simulink model "AN_Simulink_Model_v1"  (R2019b)
settings: Solver=VariableStepAuto  StartTime=0.0  StopTime=testtime  RelTol=1e-3
InitFcn:
  | AN_InitFcn_Callback
StopFcn:
  | AN_StopFcn_Callback
values from neighbouring files (symbols this model uses):
  C1initphase = C1initphase + atan(CF/(-rzero))-atan((CF-pimag(2*i-1))/(-preal(2*i-1)))-atan((CF+pimag(2*i-1))/(-preal(2*i-1)))    [AN_Get_Model_Parameters.m]
  C1slope = 0.1    [AN_Get_Model_Parameters.m]
  C2slope = 0.2    [AN_Get_Model_Parameters.m]
  CF = 2*pi*cf    [AN_Get_Model_Parameters.m]
  cf = 1000    [AN_Set_Model_Parameters.m]
  cihc = 1    [AN_Set_Model_Parameters.m]
  fs_bilinear = 2*pi*cf/tan(2*pi*cf*tdres/2)    [AN_Get_Model_Parameters.m]
  ihcasym = 3.0    (= 3)    [AN_Get_Model_Parameters.m]
  IHCLPcoeffs = [  gainihc*c2LPihc gainihc*c2LPihc 0 1 -c1LPihc 0 ... (first row only)    [AN_Get_Model_Parameters.m]
  MEcoeffs = [m14*m11 m15*m11 m16*m11 1 m12*m11 m13*m11; m24*m21 m25*m21 m26*m21 1 m22*m21 m23*m21; m34*m31 m35*m31 m36*m31 1 m32*m31 m33*m31]    [AN_Get_Model_Parameters.m]
  MEscale = 1/megainmax    (= 0.5)    [AN_Get_Model_Parameters.m]
  norm_gainc1 = single(norm_gainc1)    [AN_Get_Model_Parameters.m]
  order_of_zero = half_order_pole    (= 5)    [AN_Get_Model_Parameters.m]
  pimag = zeros(11,1)    [AN_Get_Model_Parameters.m]
  preal = zeros(11,1)    [AN_Get_Model_Parameters.m]
  strength = (20.0e6)/(10^(corner/20))    (= 2000)    [AN_Get_Model_Parameters.m]
  tauc1 = 0.003    [AN_Get_Model_Parameters.m]
  tdres = 1/Fs    (= 2.08333333333e-05)    [AN_Set_Model_Parameters.m]
undefined symbols (not defined in the file or in its folder): bmTaumax, C2coeffs, norm_gainc2
libraries: simulink x5, dspsrcs4 x1
settings Model: NumberOfSteps=50  Creator=mblun  LastModifiedBy=t96f346
settings OptimizationCC: BlockReduction=off  ConditionallyExecuteInputs=off  DefaultParameterBehavior=Inlined
settings DebuggingCC: AlgebraicLoopMsg=error  UnderSpecifiedDimensionMsg=warning
settings HardwareCC: ProdBitPerPointer=32  ProdBitPerSizeT=32  ProdBitPerPtrDiffT=32  ProdLargestAtomicFloat=None  ProdIntDivRoundTo=Undefined  ProdEndianess=Unspecified  ProdWordSize=32  ProdHWDeviceType=ASIC/FPGA->ASIC/FPGA  TargetBitPerPointer=64  TargetBitPerSizeT=64  TargetBitPerPtrDiffT=64  TargetLongLongMode=on  TargetIntDivRoundTo=Zero  TargetEndianess=LittleEndian  TargetWordSize=64  TargetHWDeviceType=Custom Processor->MATLAB Host Computer  ProdEqTarget=off
settings SFSimCC: CustomCodeUndefinedFunction=UseInterfaceOnly

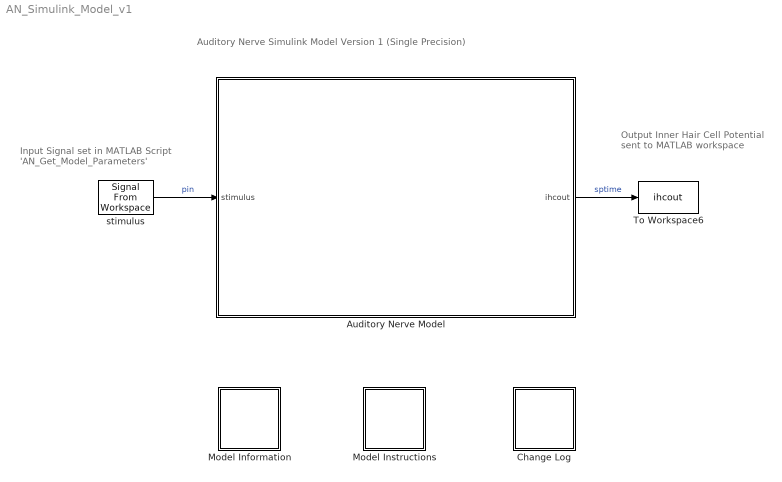
== system AN_Simulink_Model_v1 ==
  note: Input Signal set in MATLAB Script 'AN_Get_Model_Parameters'
  note: Auditory Nerve Simulink Model Version 1 (Single Precision)
  note: Output Inner Hair Cell Potential sent to MATLAB workspace
  Auditory Nerve Model : Subsystem
  Change Log : Subsystem
  Model Information : Subsystem
  Model Instructions : Subsystem
  To Workspace6 : ToWorkspace  VariableName=ihcout  SampleTime=-1
      settings: Save2DSignal=2-D array (concatenate along first dimension)
  "stimulus " : dspsrcs4/Signal From Workspace  X=RxSignal  Ts=tdres  nsamps=1  OutputAfterFinalValue=Setting to zero  ignoreOrWarnInputAndFrameLengths=off  OutputFrames=off
  wires:
  Auditory Nerve Model/1(ihcout) -> To Workspace6/1  "sptime"
  "stimulus "/1 -> Auditory Nerve Model/1(stimulus)  "pin"

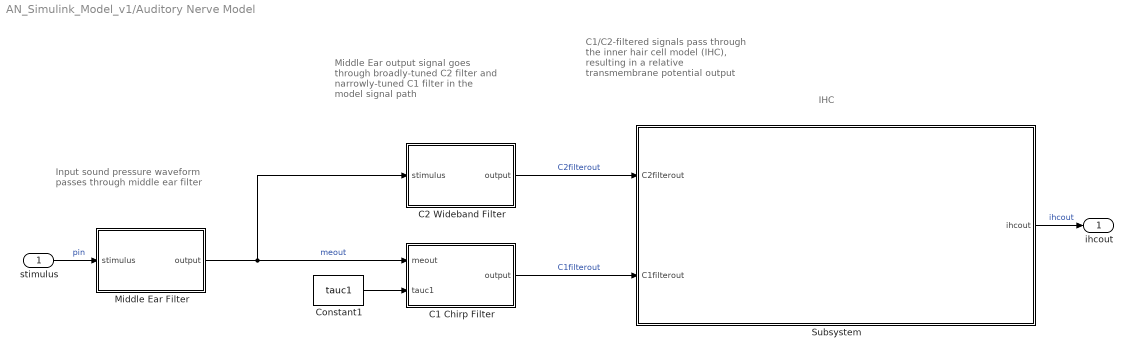
== system AN_Simulink_Model_v1/Auditory Nerve Model ==
  note: IHC
  note: Input sound pressure waveform passes through middle ear filter
  note: Middle Ear output signal goes through broadly-tuned C2 filter and narrowly-tuned C1 filter in the model signal path
  note: C1/C2-filtered signals pass through the inner hair cell model (IHC), resulting in a relative transmembrane potential output
  stimulus : Inport
  C1 Chirp Filter : Subsystem
  C2 Wideband Filter : Subsystem
  Constant1 : Constant  Value=tauc1  OutDataTypeStr=single  SampleTime=-1
  Middle Ear Filter : Subsystem
  Subsystem : Subsystem
  ihcout : Outport  VectorParamsAs1DForOutWhenUnconnected=off
  wires:
  Middle Ear Filter/1(output) -> C1 Chirp Filter/1(meout), C2 Wideband Filter/1(stimulus)  "meout"
  stimulus/1 -> Middle Ear Filter/1(stimulus)  "pin"
  C1 Chirp Filter/1(output) -> Subsystem/2(C1filterout)  "C1filterout"
  Subsystem/1(ihcout) -> ihcout/1  "ihcout"
  C2 Wideband Filter/1(output) -> Subsystem/1(C2filterout)  "C2filterout"
  Constant1/1 -> C1 Chirp Filter/2(tauc1)

== system AN_Simulink_Model_v1/Change Log ==
  Change Log : simulink/Model-Wide Utilities/Model Info  Frame=on  DisplayStringWithTags=|  HorizontalTextAlignment=Left  LeftAlignmentValue=0.02
      | The following is the change log for the AN Simulink Model. Any major version changes should be 
      | documented and summarized below.
      | 
      | ------------------------------------------------------------------------------------------------------------------------------------
      | 
      | Version 1:
      | 	
      | 	- First Draft Version of Simulink Model by Matthew Blunt --- 08/07/2019
      | 
      | ------------------------------------------------------------------------------------------------------------------------------------
      | 
      | (Next Version Here)
      | 
      | 	- (Details and Changes Here)

== system AN_Simulink_Model_v1/Model Information ==
  "Model Information " : simulink/Model-Wide Utilities/Model Info  Frame=on  DisplayStringWithTags=|  HorizontalTextAlignment=Left  LeftAlignmentValue=0.02
      | Model Name: AN_Simulink_Model_v1
      | Created By: Matthew Blunt
      | Last Modification Date: 08/07/2019
      | Most Recently Modified By: Matthew Blunt
      | Model Version: 1
      | 
      | ------------------------------------------------------------------------------------------------------------------------------------
      | 
      | Description: This is a sample-based auditory nerve Simulink model, designed to closely replicate the 
      | auditory nerve model presented in the following publication:
      | 
      | 			Bruce, I.C., Erfani, Y., and Zilany, M.S.A. (2018). "A Phenomenological
      | 			model of the synapse between the inner hair cell and auditory nerve: 
      | 			Implications of limited neurotransmitter release sites," to appear in
      | 			Hearing Research. (Special Issue on "Computational Models in Hearing".)
      | 
      | It is important to also recognize the previous iterations of the phenomenological auditory 
      | nerve model, as they served as additional references during the design of the Simulink model.
      | 
      | ------------------------------------------------------------------------------------------------------------------------------------
      | 
      | This software was developed in conjunction with Flat Earth Inc
      | 
      | Copyright 2019 Flat Earth Inc
      | 
      | THE SOFTWARE IS PROVIDED "AS IS", WITHOUT WARRANTY OF ANY KIND, EXPRESS OR
      | IMPLIED, INCLUDING BUT NOT LIMITED TO THE WARRANTIES OF MERCHANTABILITY,
      | FITNESS FOR A PARTICULAR PURPOSE AND NONINFRINGEMENT. IN NO EVENT SHALL
      | THE AUTHORS OR COPYRIGHT HOLDERS BE LIABLE FOR ANY CLAIM, DAMAGES OR
      | OTHER LIABILITY, WHETHER IN AN ACTION OF CONTRACT, TORT OR OTHERWISE,
      | ARISING FROM, OUT OF OR IN CONNECTION WITH THE SOFTWARE OR THE USE OR
      | OTHER DEALINGS IN THE SOFTWARE.
      | 
      |    		Matthew Blunt
      |   		 Flat Earth Inc
      |    		985 Technology Blvd
      |    		Bozeman, MT 59718
      |    		support@flatearthinc.com

== system AN_Simulink_Model_v1/Model Instructions ==
  "Model Instructions " : simulink/Model-Wide Utilities/Model Info  Frame=on  DisplayStringWithTags=|  HorizontalTextAlignment=Left  LeftAlignmentValue=0.02
      | The following is a full set of instructions outlining the necessary steps to be taken in order to run the 
      | AN Simulink Model. Instructions can also be found in the readme file found in the
      | AN_Simulink_Model_v1_Doubles folder.
      | 
      | ------------------------------------------------------------------------------------------------------------------------------------
      | 
      | ** Quick Start Instructions **
      | 
      | If the user desires to simply run the model as is, refer to the Quick Start
      | Instructions pdf, which gives a quick visual tutorial on running the Auditory
      | Nerve Simulink Model.
      | 
      | ------------------------------------------------------------------------------------------------------------------------------------
      | 
      | ** Modify Model Instructions **
      | 
      | If the user desires to make modifications to the model before runtime,
      | refer to the Modify Model Instructions pdf, which gives a quick visual
      | tutorial on modifying the Auditory Nerve Simulink Model.
      | 
      | ------------------------------------------------------------------------------------------------------------------------------------
      | 
      | ** Verify Model Instructions **
      | 
      | If the user desires to verify model functionality against the original 
      | model source code, instructions are listed below, as well as in the readme.txt file
      | 
      | 1. Make sure MATLAB R2019a and a compatible C compiler are downloaded on the
      | machine the model will be running on. The C compiler is needed for C functions
      | used in the test/verification process. The compiler used for testing was the
      | MinGW-w64 C/C++ Compiler. This can be easily accessed for free in the Add-On
      | Explorer found in the MATLAB home tab.
      | 
      | 2. Open the AN_Simulink_Model_v1_Doubles folder in MATLAB. This is necessary in
      | order for the Simulink model to interact with MATLAB.
      | 
      | 3. Edit model parameters, if necessary. This can be done by adjusting the
      | overall model parameters set in the AN_Set_Model_Parameters script, or adjusting
      | other parameters in the AN_Get_Model_Parameters script. Both scripts are found
      | in the AN_Simulink_Model_v1_Doubles folder.
      | 
      | 4. Set the 'verificationflag' boolean to 'true' in the AN_Set_Model_Parameters
      | script. This enables the model to run the comparison C/MATLAB source functions
      | which are compared to the Simulink Model.
      | 
      | 5. Run the model. This is done by simply clicking the green 'Run' button
      | located at the top panel of Simulink. In addition, the model can be stepped
      | through in increments, using the 'Step Through' button to the right of the
      | 'Run' button.

== system AN_Simulink_Model_v1/Auditory Nerve Model/C1 Chirp Filter ==
  note: C1 Chirp Filter:
      |
      | Inputs : ME Filtered Signal (meout)
      | C1 Coefficients (a&b)
      | Normalizing Gain (norm_gain)
      |
      | Output : C1 Filtered Signal (c1filterout)
      |
      | - 10th Order IIR Bandpass Filter
      |
      | - Coefficients are determined in previous Get C1 Coefficients block
      |
      | - Implemented w/ Simulink biquad block
  note: Get C1 Coefficients
      |
      | Input : Pole-Shifting Feedback Parameter (rsigma)
      |
      | Outputs : C1 Coefficients (a&b)
      | Normalizing Gain (norm_gain)
      |
      | - Consists of various calculations to shift continuous-time pole locations according to rsigma feedback, then apply a bilinear transformation to bring the poles to the digital space before finding the coefficients for the C1 filter
  note: Calculate C1 Filter Output
      |
      | - Simply scale the output by cihc
  note: Calculate Pole-Shifting Parameter rsigma
      |
      | Input : C1 Feedback Time Constant (tauc1)
      |
      | Outputs : Pole-Shifting Parameter rsigma
      |
      | - Simple calculation to find rsigma from time constant feedback input
  meout : Inport
  tauc1 : Inport  Port=2
  C1 FIlter : Subsystem
  Calculate C1filterout : Subsystem
  Calculate rsigma : Subsystem
  Get C1 Coefficients : Subsystem
  output : Outport  VectorParamsAs1DForOutWhenUnconnected=off
  wires:
  meout/1 -> C1 FIlter/1(meout)
  C1 FIlter/1(Out1) -> Calculate C1filterout/1(C1filterouttmp)  "c1filterouttmp"
  Get C1 Coefficients/1(b0(5)) -> C1 FIlter/2(b0(5))
  Get C1 Coefficients/2(b0(3)) -> C1 FIlter/3(b0(3))
  Get C1 Coefficients/3(b0(1)) -> C1 FIlter/4(b0(1))
  Get C1 Coefficients/4(b1(5)) -> C1 FIlter/5(b1(5))
  Get C1 Coefficients/5(b1(3)) -> C1 FIlter/6(b1(3))
  Get C1 Coefficients/6(b1(1)) -> C1 FIlter/7(b1(1))
  Get C1 Coefficients/7(b2(5)) -> C1 FIlter/8(b2(5))
  Get C1 Coefficients/8(b2(3)) -> C1 FIlter/9(b2(3))
  Get C1 Coefficients/9(b2(1)) -> C1 FIlter/10(b2(1))
  Get C1 Coefficients/10(a2(5)) -> C1 FIlter/11(a2(5))
  Get C1 Coefficients/11(a2(3)) -> C1 FIlter/12(a2(3))
  Get C1 Coefficients/12(a2(1)) -> C1 FIlter/13(a2(1))
  Get C1 Coefficients/13(a1(1)) -> C1 FIlter/14(a1(1))
  Get C1 Coefficients/14(a1(3)) -> C1 FIlter/15(a1(3))
  Get C1 Coefficients/15(a1(5)) -> C1 FIlter/16(a1(5))
  Calculate C1filterout/1(C1filterout) -> output/1  "C1filterout"
  Calculate rsigma/1(rsigma) -> Get C1 Coefficients/1(rsigma)  "rsigma"
  tauc1/1 -> Calculate rsigma/1(tauc1)  "tauc1"

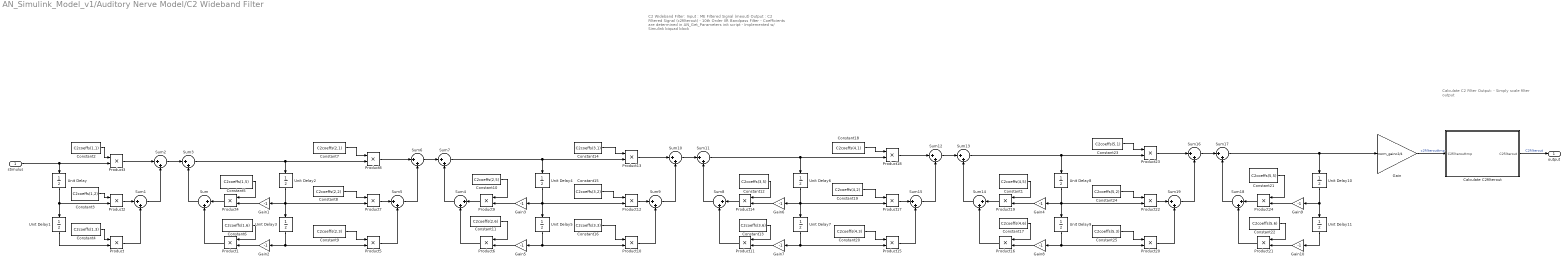
== system AN_Simulink_Model_v1/Auditory Nerve Model/C2 Wideband Filter ==
  note: C2 Wideband Filter:
      |
      | Input : ME Filtered Signal (meout)
      |
      | Output : C2 Filtered Signal (c2filterout)
      |
      | - 10th Order IIR Bandpass Filter
      |
      | - Coefficients are determined in AN_Get_Parameters init script
      |
      | - Implemented w/ Simulink biquad block
  note: Calculate C2 Filter Output:
      |
      | - Simply scale filter output
  stimulus : Inport
  Calculate C2filterout : Subsystem
  Constant1 : Constant  Value=C2coeffs(4,5)  OutDataTypeStr=single  SampleTime=-1
  Constant10 : Constant  Value=C2coeffs(2,5)  OutDataTypeStr=single  SampleTime=-1
  Constant11 : Constant  Value=C2coeffs(2,6)  OutDataTypeStr=single  SampleTime=-1
  Constant12 : Constant  Value=C2coeffs(3,5)  OutDataTypeStr=single  SampleTime=-1
  Constant13 : Constant  Value=C2coeffs(3,6)  OutDataTypeStr=single  SampleTime=-1
  Constant14 : Constant  Value=C2coeffs(3,1)  OutDataTypeStr=single  SampleTime=-1
  Constant15 : Constant  Value=C2coeffs(3,2)  OutDataTypeStr=single  SampleTime=-1
  Constant16 : Constant  Value=C2coeffs(3,3)  OutDataTypeStr=single  SampleTime=-1
  Constant17 : Constant  Value=C2coeffs(4,6)  OutDataTypeStr=single  SampleTime=-1
  Constant18 : Constant  Value=C2coeffs(4,1)  OutDataTypeStr=single  SampleTime=-1
  Constant19 : Constant  Value=C2coeffs(4,2)  OutDataTypeStr=single  SampleTime=-1
  Constant2 : Constant  Value=C2coeffs(1,1)  OutDataTypeStr=single  SampleTime=-1
  Constant20 : Constant  Value=C2coeffs(4,3)  OutDataTypeStr=single  SampleTime=-1
  Constant21 : Constant  Value=C2coeffs(5,5)  OutDataTypeStr=single  SampleTime=-1
  Constant22 : Constant  Value=C2coeffs(5,6)  OutDataTypeStr=single  SampleTime=-1
  Constant23 : Constant  Value=C2coeffs(5,1)  OutDataTypeStr=single  SampleTime=-1
  Constant24 : Constant  Value=C2coeffs(5,2)  OutDataTypeStr=single  SampleTime=-1
  Constant25 : Constant  Value=C2coeffs(5,3)  OutDataTypeStr=single  SampleTime=-1
  Constant3 : Constant  Value=C2coeffs(1,2)  OutDataTypeStr=single  SampleTime=-1
  Constant4 : Constant  Value=C2coeffs(1,3)  OutDataTypeStr=single  SampleTime=-1
  Constant5 : Constant  Value=C2coeffs(1,5)  OutDataTypeStr=single  SampleTime=-1
  Constant6 : Constant  Value=C2coeffs(1,6)  OutDataTypeStr=single  SampleTime=-1
  Constant7 : Constant  Value=C2coeffs(2,1)  OutDataTypeStr=single  SampleTime=-1
  Constant8 : Constant  Value=C2coeffs(2,2)  OutDataTypeStr=single  SampleTime=-1
  Constant9 : Constant  Value=C2coeffs(2,3)  OutDataTypeStr=single  SampleTime=-1
  Gain : Gain  Gain=norm_gainc2/4
  Gain{1..10} (10 alike) : Gain  Gain=-1
  Product{,1..24} (25 alike) : Product
  Sum{,1..19} (20 alike) : Sum  Inputs=|++
  Unit Delay{,1..11} (12 alike) : UnitDelay  SampleTime=-1  HasFrameUpgradeWarning=on
  output : Outport  VectorParamsAs1DForOutWhenUnconnected=off
  wires:
  Sum17/1 -> Gain/1, Unit Delay10/1
  Gain/1 -> Calculate C2filterout/1(C2filterouttmp)  "c2filterouttmp"
  Calculate C2filterout/1(C2filterout) -> output/1  "C2filterout"
  Sum8/1 -> Sum11/2
  Gain4/1 -> Product19/2
  Sum10/1 -> Sum11/1
  Constant15/1 -> Product12/1
  Unit Delay10/1 -> Unit Delay11/1, Gain9/1
  Product17/1 -> Sum15/1
  Constant6/1 -> Product1/1
  Constant22/1 -> Product21/1
  Unit Delay6/1 -> Product17/2, Unit Delay7/1, Gain6/1
  Sum11/1 -> Unit Delay6/1, Product18/2
  Sum6/1 -> Sum7/1
  Product18/1 -> Sum12/1
  Product23/1 -> Sum16/1
  Constant21/1 -> Product24/1
  Unit Delay8/1 -> Product22/2, Unit Delay9/1, Gain4/1
  Gain3/1 -> Product9/2
  Constant19/1 -> Product17/1
  Product/1 -> Sum1/2
  Unit Delay/1 -> Unit Delay1/1, Product2/2
  Product20/1 -> Sum19/2
  Sum3/1 -> Unit Delay2/1, Product8/2
  Gain2/1 -> Product1/2
  Constant5/1 -> Product4/1
  Constant12/1 -> Product14/1
  Sum15/1 -> Sum12/2
  Sum4/1 -> Sum7/2
  Constant14/1 -> Product13/1
  Constant10/1 -> Product9/1
  Sum14/1 -> Sum13/2
  Unit Delay11/1 -> Gain10/1
  Product13/1 -> Sum10/1
  Product4/1 -> Sum/1
  Gain10/1 -> Product21/2
  Constant8/1 -> Product7/1
  Sum2/1 -> Sum3/1
  Constant4/1 -> Product/1
  Sum7/1 -> Unit Delay4/1, Product13/2
  Unit Delay7/1 -> Product15/2, Gain7/1
  Sum12/1 -> Sum13/1
  Unit Delay9/1 -> Product20/2, Gain8/1
  Product1/1 -> Sum/2
  Sum18/1 -> Sum17/2
  Sum1/1 -> Sum2/2
  Constant23/1 -> Product23/1
  Product24/1 -> Sum18/1
  Product11/1 -> Sum8/2
  Product21/1 -> Sum18/2
  Constant3/1 -> Product2/1
  Constant2/1 -> Product3/1
  Product5/1 -> Sum5/2
  Constant7/1 -> Product8/1
  Sum/1 -> Sum3/2
  Product8/1 -> Sum6/1
  Gain5/1 -> Product6/2
  Gain9/1 -> Product24/2
  Product16/1 -> Sum14/2
  Unit Delay4/1 -> Product12/2, Unit Delay5/1, Gain3/1
  Constant16/1 -> Product10/1
  Product15/1 -> Sum15/2
  Constant20/1 -> Product15/1
  stimulus/1 -> Product3/2, Unit Delay/1
  Product3/1 -> Sum2/1
  Unit Delay1/1 -> Product/2
  Product2/1 -> Sum1/1
  Constant24/1 -> Product22/1
  Gain8/1 -> Product16/2
  Sum16/1 -> Sum17/1
  Unit Delay3/1 -> Product5/2, Gain2/1
  Constant9/1 -> Product5/1
  Product6/1 -> Sum4/2
  Sum19/1 -> Sum16/2
  Gain1/1 -> Product4/2
  Product10/1 -> Sum9/2
  Product22/1 -> Sum19/1
  Unit Delay5/1 -> Product10/2, Gain5/1
  Unit Delay2/1 -> Product7/2, Unit Delay3/1, Gain1/1
  Product9/1 -> Sum4/1
  Gain6/1 -> Product14/2
  Constant1/1 -> Product19/1
  Constant17/1 -> Product16/1
  Product14/1 -> Sum8/1
  Product19/1 -> Sum14/1
  Product7/1 -> Sum5/1
  Constant13/1 -> Product11/1
  Constant25/1 -> Product20/1
  Gain7/1 -> Product11/2
  Constant11/1 -> Product6/1
  Sum5/1 -> Sum6/2
  Constant18/1 -> Product18/1
  Sum13/1 -> Unit Delay8/1, Product23/2
  Sum9/1 -> Sum10/2
  Product12/1 -> Sum9/1

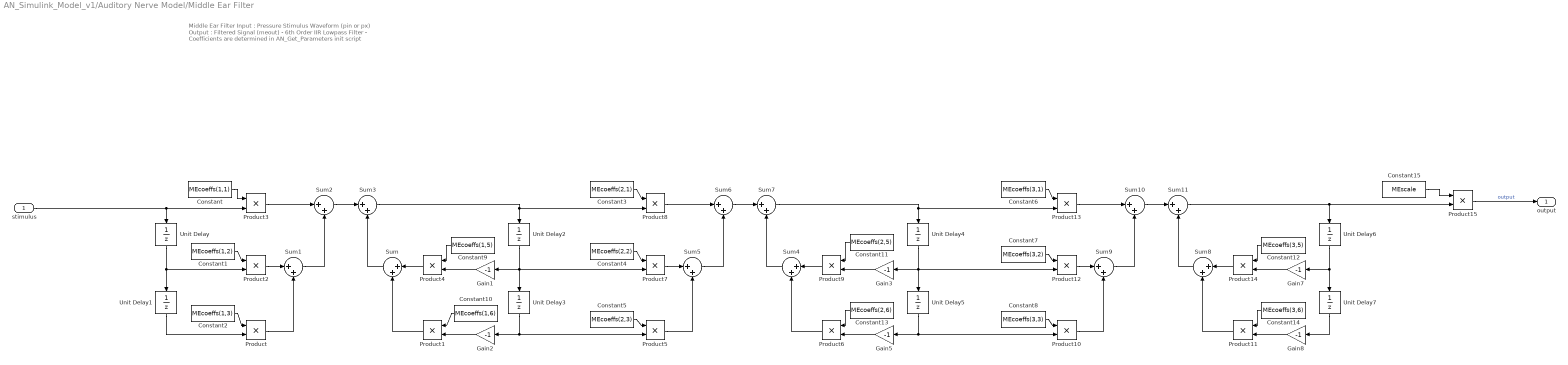
== system AN_Simulink_Model_v1/Auditory Nerve Model/Middle Ear Filter ==
  note: Middle Ear Filter
      |
      | Input : Pressure Stimulus Waveform (pin or px)
      |
      | Output : Filtered Signal (meout)
      |
      | - 6th Order IIR Lowpass Filter
      |
      | - Coefficients are determined in AN_Get_Parameters init script
  stimulus : Inport
  Constant : Constant  Value=MEcoeffs(1,1)  OutDataTypeStr=single  SampleTime=-1
  Constant1 : Constant  Value=MEcoeffs(1,2)  OutDataTypeStr=single  SampleTime=-1
  Constant10 : Constant  Value=MEcoeffs(1,6)  OutDataTypeStr=single  SampleTime=-1
  Constant11 : Constant  Value=MEcoeffs(2,5)  OutDataTypeStr=single  SampleTime=-1
  Constant12 : Constant  Value=MEcoeffs(3,5)  OutDataTypeStr=single  SampleTime=-1
  Constant13 : Constant  Value=MEcoeffs(2,6)  OutDataTypeStr=single  SampleTime=-1
  Constant14 : Constant  Value=MEcoeffs(3,6)  OutDataTypeStr=single  SampleTime=-1
  Constant15 : Constant  Value=MEscale  OutDataTypeStr=single  SampleTime=-1
  Constant2 : Constant  Value=MEcoeffs(1,3)  OutDataTypeStr=single  SampleTime=-1
  Constant3 : Constant  Value=MEcoeffs(2,1)  OutDataTypeStr=single  SampleTime=-1
  Constant4 : Constant  Value=MEcoeffs(2,2)  OutDataTypeStr=single  SampleTime=-1
  Constant5 : Constant  Value=MEcoeffs(2,3)  OutDataTypeStr=single  SampleTime=-1
  Constant6 : Constant  Value=MEcoeffs(3,1)  OutDataTypeStr=single  SampleTime=-1
  Constant7 : Constant  Value=MEcoeffs(3,2)  OutDataTypeStr=single  SampleTime=-1
  Constant8 : Constant  Value=MEcoeffs(3,3)  OutDataTypeStr=single  SampleTime=-1
  Constant9 : Constant  Value=MEcoeffs(1,5)  OutDataTypeStr=single  SampleTime=-1
  Gain{1..3,5,7..8} (6 alike) : Gain  Gain=-1
  Product{,1..15} (16 alike) : Product
  Sum{,1..11} (12 alike) : Sum  Inputs=|++
  Unit Delay{,1..7} (8 alike) : UnitDelay  SampleTime=-1  HasFrameUpgradeWarning=on
  output : Outport  VectorParamsAs1DForOutWhenUnconnected=off
  wires:
  Product15/1 -> output/1  "output"
  Constant13/1 -> Product6/1
  Constant6/1 -> Product13/1
  Gain8/1 -> Product11/2
  Sum8/1 -> Sum11/2
  Constant11/1 -> Product9/1
  Sum9/1 -> Sum10/2
  Constant12/1 -> Product14/1
  Constant15/1 -> Product15/1
  Constant14/1 -> Product11/1
  Unit Delay5/1 -> Product10/2, Gain5/1
  Sum4/1 -> Sum7/2
  Unit Delay/1 -> Unit Delay1/1, Product2/2
  Constant4/1 -> Product7/1
  Unit Delay7/1 -> Gain8/1
  Constant8/1 -> Product10/1
  Sum/1 -> Sum3/2
  Constant2/1 -> Product/1
  Constant7/1 -> Product12/1
  Product10/1 -> Sum9/2
  Constant/1 -> Product3/1
  Sum7/1 -> Product13/2, Unit Delay4/1
  Product1/1 -> Sum/2
  Product7/1 -> Sum5/1
  Constant1/1 -> Product2/1
  Unit Delay1/1 -> Product/2
  Product14/1 -> Sum8/1
  Gain7/1 -> Product14/2
  Sum3/1 -> Product8/2, Unit Delay2/1
  Product11/1 -> Sum8/2
  Sum5/1 -> Sum6/2
  stimulus/1 -> Product3/2, Unit Delay/1
  Sum1/1 -> Sum2/2
  Product6/1 -> Sum4/2
  Product12/1 -> Sum9/1
  Product5/1 -> Sum5/2
  Product3/1 -> Sum2/1
  Product2/1 -> Sum1/1
  Product9/1 -> Sum4/1
  Unit Delay6/1 -> Unit Delay7/1, Gain7/1
  Unit Delay3/1 -> Product5/2, Gain2/1
  Product13/1 -> Sum10/1
  Product4/1 -> Sum/1
  Unit Delay4/1 -> Product12/2, Unit Delay5/1, Gain3/1
  Product/1 -> Sum1/2
  Constant5/1 -> Product5/1
  Sum11/1 -> Product15/2, Unit Delay6/1
  Unit Delay2/1 -> Product7/2, Unit Delay3/1, Gain1/1
  Product8/1 -> Sum6/1
  Gain2/1 -> Product1/2
  Sum10/1 -> Sum11/1
  Sum6/1 -> Sum7/1
  Constant9/1 -> Product4/1
  Constant10/1 -> Product1/1
  Sum2/1 -> Sum3/1
  Gain1/1 -> Product4/2
  Gain3/1 -> Product9/2
  Gain5/1 -> Product6/2
  Constant3/1 -> Product8/1

== system AN_Simulink_Model_v1/Auditory Nerve Model/Subsystem ==
  note: Sum Nonlinear Function Outputs
  note: IHC C2 Nonlinear Logarithmic Transduction Function
      |
      | Input : C2 Filtered Signal (c2filterout)
      |
      | Output : C2 Transduction Function Output (c2vihctmp)
  note: IHC C1 Nonlinear Logarithmic Transduction Function
      |
      | Input : C1 Filtered Signal (c1filterout)
      |
      | Output : C1 Transduction Function Output (c1vihctmp)
  note: IHC Lowpass Filter
      |
      | Input : Sum of C1 and C2 Nonlinear Outputs (ihcnonlinout)
      |
      | Output : IHC Output (ihcout)
      |
      | - 7th Order IIR Lowpass Filter
      |
      | - Implemented using Simulink biquad
  C2filterout : Inport
  C1filterout : Inport  Port=2
  IHC C1 NL Logarithmic Function : Subsystem
  IHC C2 NL Logarithmic Function : Subsystem
  IHC LP Filter : Subsystem
  Sum1 : Sum  Inputs=|++
  ihcout : Outport  VectorParamsAs1DForOutWhenUnconnected=off
  wires:
  IHC C2 NL Logarithmic Function/1(output) -> Sum1/1  "c2vihctmp"
  IHC C1 NL Logarithmic Function/1(output) -> Sum1/2  "c1vihctmp"
  C1filterout/1 -> IHC C1 NL Logarithmic Function/1(stimulus)  "c1filterout"
  IHC LP Filter/1(output) -> ihcout/1  "ihcout"
  Sum1/1 -> IHC LP Filter/1(stimulus)  "ihcnonlinout"
  C2filterout/1 -> IHC C2 NL Logarithmic Function/1(stimulus)  "c2filterout"

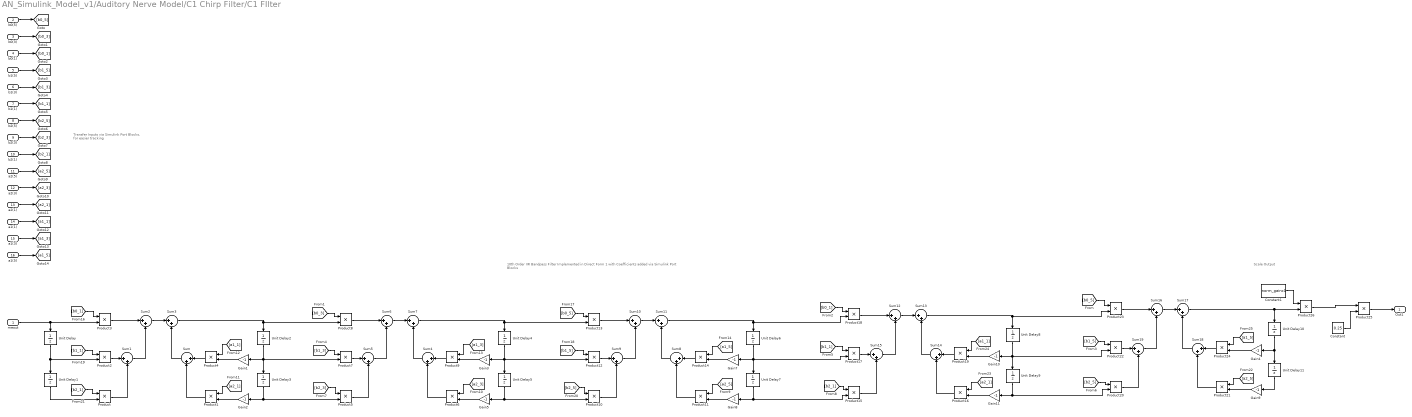
== system AN_Simulink_Model_v1/Auditory Nerve Model/C1 Chirp Filter/C1 FIlter ==
  note: Transfer Inputs via Simulink Port Blocks, for easier tracking
  note: 10th Order IIR Bandpass Filter Implemented in Direct Form 1 with Coefficients added via Simulink Port Blocks
  note: Scale Output
  meout : Inport
  b0(5) : Inport  Port=2
  b0(3) : Inport  Port=3
  b0(1) : Inport  Port=4
  b1(5) : Inport  Port=5
  b1(3) : Inport  Port=6
  b1(1) : Inport  Port=7
  b2(5) : Inport  Port=8
  b2(3) : Inport  Port=9
  b2(1) : Inport  Port=10
  a2(5) : Inport  Port=11
  a2(3) : Inport  Port=12
  a2(1) : Inport  Port=13
  a1(1) : Inport  Port=14
  a1(3) : Inport  Port=15
  a1(5) : Inport  Port=16
  Constant : Constant  Value=0.25  OutDataTypeStr=single  SampleTime=-1
  Constant1 : Constant  Value=norm_gainc1  OutDataTypeStr=single  SampleTime=-1
  Gain{1..5,7..11} (10 alike) : Gain  Gain=-1
  Product{,1..24} (25 alike) : Product
  Product25 : Product  OutDataTypeStr=single
  Product26 : Product  OutDataTypeStr=single
  Sum{,1..19} (20 alike) : Sum  Inputs=|++
  Unit Delay{,1..11} (12 alike) : UnitDelay  SampleTime=-1  HasFrameUpgradeWarning=on
  Out1 : Outport  VectorParamsAs1DForOutWhenUnconnected=off
  wires:
  [a1_5] -> Product14/1
  Product15/1 -> Sum15/2
  Product16/1 -> Sum14/2
  Sum5/1 -> Sum6/2
  Sum15/1 -> Sum12/2
  Unit Delay2/1 -> Product7/2, Unit Delay3/1, Gain1/1
  Unit Delay6/1 -> Product17/2, Unit Delay7/1, Gain7/1
  [b1_3] -> Product7/1
  Sum1/1 -> Sum2/2
  [b0_1] -> Product3/1
  Product4/1 -> Sum/1
  Unit Delay8/1 -> Product22/2, Unit Delay9/1, Gain10/1
  Product12/1 -> Sum9/1
  Sum17/1 -> Product26/2, Unit Delay10/1
  Product3/1 -> Sum2/1
  [b2_3] -> Product5/1
  Sum7/1 -> Product13/2, Unit Delay4/1
  [a2_1] -> Product1/1
  [b2_1] -> Product/1
  Product24/1 -> Sum18/1
  Unit Delay3/1 -> Product5/2, Gain2/1
  Product5/1 -> Sum5/2
  Unit Delay4/1 -> Product12/2, Unit Delay5/1, Gain3/1
  Sum13/1 -> Product23/2, Unit Delay8/1
  Sum3/1 -> Product8/2, Unit Delay2/1
  Sum4/1 -> Sum7/2
  Product19/1 -> Sum14/1
  Product7/1 -> Sum5/1
  Product10/1 -> Sum9/2
  Product20/1 -> Sum19/2
  [a1_5] -> Product24/1
  Sum6/1 -> Sum7/1
  [b0_5] -> Product13/1
  [a1_3] -> Product9/1
  Product22/1 -> Sum19/1
  Product8/1 -> Sum6/1
  meout/1 -> Product3/2, Unit Delay/1
  Product2/1 -> Sum1/1
  Sum11/1 -> Product18/2, Unit Delay6/1
  Unit Delay5/1 -> Product10/2, Gain5/1
  [b1_5] -> Product12/1
  Sum2/1 -> Sum3/1
  Product11/1 -> Sum8/2
  Sum19/1 -> Sum16/2
  [b2_5] -> Product20/1
  Product14/1 -> Sum8/1
  Product18/1 -> Sum12/1
  Sum8/1 -> Sum11/2
  [b0_3] -> Product8/1
  Sum12/1 -> Sum13/1
  [b0_5] -> Product23/1
  [b0_1] -> Product18/1
  [a1_1] -> Product19/1
  [a2_5] -> Product21/1
  Unit Delay/1 -> Unit Delay1/1, Product2/2
  Product17/1 -> Sum15/1
  Unit Delay7/1 -> Product15/2, Gain8/1
  Unit Delay10/1 -> Unit Delay11/1, Gain4/1
  [a2_5] -> Product11/1
  Unit Delay11/1 -> Gain9/1
  Product25/1 -> Out1/1
  Product23/1 -> Sum16/1
  Product9/1 -> Sum4/1
  [b1_1] -> Product17/1
  Product13/1 -> Sum10/1
  Product6/1 -> Sum4/2
  Sum9/1 -> Sum10/2
  Sum16/1 -> Sum17/1
  Product21/1 -> Sum18/2
  [b1_1] -> Product2/1
  Sum18/1 -> Sum17/2
  [b1_5] -> Product22/1
  [a2_1] -> Product16/1
  [a2_3] -> Product6/1
  Sum10/1 -> Sum11/1
  [b2_5] -> Product10/1
  [b2_1] -> Product15/1
  Product/1 -> Sum1/2
  Unit Delay9/1 -> Product20/2, Gain11/1
  Sum14/1 -> Sum13/2
  [a1_1] -> Product4/1
  Sum/1 -> Sum3/2
  Unit Delay1/1 -> Product/2
  Product1/1 -> Sum/2
  b0(5)/1 -> [b0_5]
  b0(3)/1 -> [b0_3]
  b0(1)/1 -> [b0_1]
  b1(5)/1 -> [b1_5]
  b1(3)/1 -> [b1_3]
  b1(1)/1 -> [b1_1]
  b2(5)/1 -> [b2_5]
  b2(3)/1 -> [b2_3]
  b2(1)/1 -> [b2_1]
  a2(5)/1 -> [a2_5]
  a2(3)/1 -> [a2_3]
  a2(1)/1 -> [a2_1]
  a1(1)/1 -> [a1_1]
  a1(3)/1 -> [a1_3]
  a1(5)/1 -> [a1_5]
  Gain1/1 -> Product4/2
  Gain2/1 -> Product1/2
  Gain3/1 -> Product9/2
  Gain5/1 -> Product6/2
  Gain7/1 -> Product14/2
  Gain8/1 -> Product11/2
  Gain10/1 -> Product19/2
  Gain11/1 -> Product16/2
  Gain4/1 -> Product24/2
  Gain9/1 -> Product21/2
  Constant/1 -> Product25/2
  Product26/1 -> Product25/1
  Constant1/1 -> Product26/1

== system AN_Simulink_Model_v1/Auditory Nerve Model/C1 Chirp Filter/Calculate C1filterout ==
  C1filterouttmp : Inport
  Gain1 : Gain  Gain=cihc
  C1filterout : Outport  VectorParamsAs1DForOutWhenUnconnected=off
  wires:
  C1filterouttmp/1 -> Gain1/1
  Gain1/1 -> C1filterout/1

== system AN_Simulink_Model_v1/Auditory Nerve Model/C1 Chirp Filter/Calculate rsigma ==
  note: Note: There are multiple HDL-friendly recipricol blocks. Use this block type for highest accuracy.
  note: Calculating rsigma using time constant feedback input
  tauc1 : Inport
  Constant2 : Constant  Value=bmTaumax  OutDataTypeStr=single  SampleTime=-1
  Reciprocal : Product  Inputs=/  SaturateOnIntegerOverflow=on  RndMeth=Zero
  Reciprocal1 : Product  Inputs=/  SaturateOnIntegerOverflow=on  RndMeth=Zero
  Subtract : Sum  Inputs=+-
  rsigma : Outport  VectorParamsAs1DForOutWhenUnconnected=off
  wires:
  tauc1/1 -> Reciprocal/1
  Constant2/1 -> Reciprocal1/1
  Reciprocal/1 -> Subtract/1
  Reciprocal1/1 -> Subtract/2
  Subtract/1 -> rsigma/1

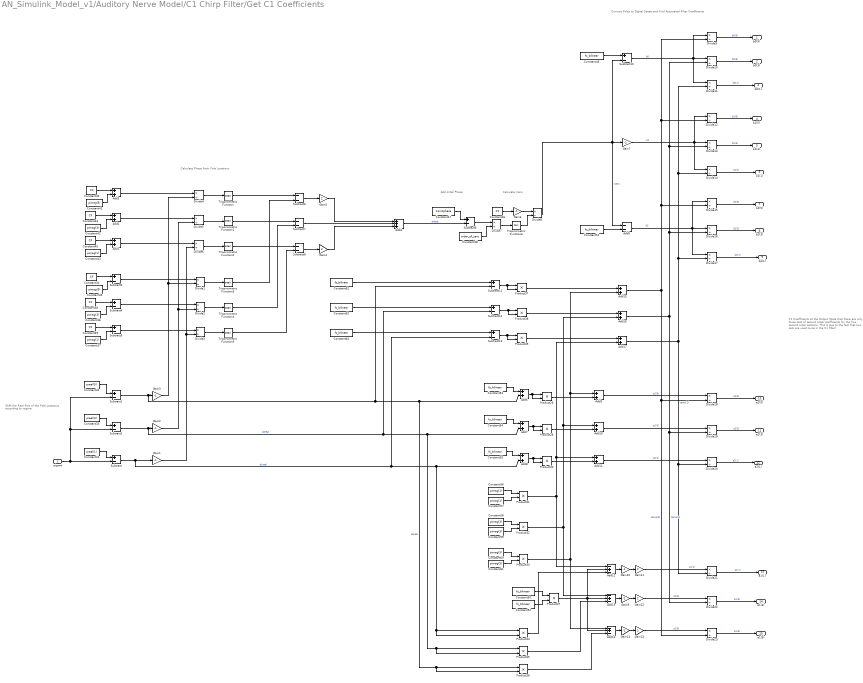
== system AN_Simulink_Model_v1/Auditory Nerve Model/C1 Chirp Filter/Get C1 Coefficients ==
  note: Calculate Phase from Pole Locations
  note: Shift the Real Part of the Pole Locations according to rsigma
  note: Add Initial Phase
  note: Calculate rzero
  note: Convert Poles to Digital Spcae and Find Associated Filter Coefficients
  note: C1 Coefficients at the Output (Note that there are only three sets of second order coefficients for the five second order sections. This is due to the fact that two sets are used twice in the C1 filter)
  rsigma : Inport
  Add{1..3,6..11,15..17} (12 alike) : Sum
  Add12 : Sum  Inputs=-+-
  Add13 : Sum  Inputs=-+-
  Add14 : Sum  Inputs=-+-
  Add4 : Sum  Inputs=+++
  Add5 : Sum  Inputs=--
  Constant31 : Constant  Value=preal(1)  OutDataTypeStr=single  SampleTime=-1
  Constant32 : Constant  Value=preal(5)  OutDataTypeStr=single  SampleTime=-1
  Constant33 : Constant  Value=preal(3)  OutDataTypeStr=single  SampleTime=-1
  Constant{34,38..40,44..46} (7 alike) : Constant  Value=CF  OutDataTypeStr=single  SampleTime=-1
  Constant{35,41,60..61} (4 alike) : Constant  Value=pimag(5)  OutDataTypeStr=single  SampleTime=-1
  Constant{36,42,58..59} (4 alike) : Constant  Value=pimag(3)  OutDataTypeStr=single  SampleTime=-1
  Constant{37,43,56..57} (4 alike) : Constant  Value=pimag(1)  OutDataTypeStr=single  SampleTime=-1
  Constant47 : Constant  Value=C1initphase  OutDataTypeStr=single  SampleTime=-1
  Constant48 : Constant  Value=order_of_zero  OutDataTypeStr=single  SampleTime=-1
  Constant{49..55,62..64} (10 alike) : Constant  Value=fs_bilinear  OutDataTypeStr=single  SampleTime=-1
  Divide{1..23} (23 alike) : Product  Inputs=*/  SaturateOnIntegerOverflow=on  RndMeth=Zero
  Gain{1..3,6,9..10,14} (7 alike) : Gain  Gain=-1
  Gain{4..5,11..13} (5 alike) : Gain  Gain=2
  Gain7 : Gain  Gain=-2
  Product{27..39} (13 alike) : Product
  Subtract{,1..5,9..13} (11 alike) : Sum  Inputs=+-
  Subtract6 : Sum  Inputs=--
  Subtract7 : Sum  Inputs=--
  Subtract8 : Sum  Inputs=--
  Trigonometric Function{,1..5} (6 alike) : Trigonometry  Operator=atan  ApproximationMethod=CORDIC
  Trigonometric Function6 : Trigonometry  Operator=tan  ApproximationMethod=CORDIC
  b0(5) : Outport  VectorParamsAs1DForOutWhenUnconnected=off
  b0(3) : Outport  Port=2  VectorParamsAs1DForOutWhenUnconnected=off
  b0(1) : Outport  Port=3  VectorParamsAs1DForOutWhenUnconnected=off
  b1(5) : Outport  Port=4  VectorParamsAs1DForOutWhenUnconnected=off
  b1(3) : Outport  Port=5  VectorParamsAs1DForOutWhenUnconnected=off
  b1(1) : Outport  Port=6  VectorParamsAs1DForOutWhenUnconnected=off
  b2(5) : Outport  Port=7  VectorParamsAs1DForOutWhenUnconnected=off
  b2(3) : Outport  Port=8  VectorParamsAs1DForOutWhenUnconnected=off
  b2(1) : Outport  Port=9  VectorParamsAs1DForOutWhenUnconnected=off
  a2(5) : Outport  Port=10  VectorParamsAs1DForOutWhenUnconnected=off
  a2(3) : Outport  Port=11  VectorParamsAs1DForOutWhenUnconnected=off
  a2(1) : Outport  Port=12  VectorParamsAs1DForOutWhenUnconnected=off
  a1(1) : Outport  Port=13  VectorParamsAs1DForOutWhenUnconnected=off
  a1(3) : Outport  Port=14  VectorParamsAs1DForOutWhenUnconnected=off
  a1(5) : Outport  Port=15  VectorParamsAs1DForOutWhenUnconnected=off
  wires:
  Add5/1 -> Divide17/1, Divide16/1, Divide15/1  "b2"
  Constant46/1 -> Gain6/1
  Divide6/1 -> Trigonometric Function2/1
  Divide18/1 -> a2(5)/1  "a2(5)"
  Subtract9/1 -> Divide7/1
  Constant33/1 -> Subtract2/1
  Add17/1 -> Divide21/2, Divide20/2, Divide17/2, Divide11/2, Divide14/2  "temp(1)"
  Product31/1 -> Add12/1, Add17/2, Add11/1
  Gain2/1 -> Divide5/2, Divide2/2
  Subtract8/1 -> Gain4/1
  rsigma/1 -> Subtract/2, Subtract1/2, Subtract2/2
  Gain1/1 -> Divide6/2, Divide3/2
  Add12/1 -> Gain10/1
  Constant52/1 -> Product27/2
  Add13/1 -> Gain9/1
  Add15/1 -> Divide23/2, Divide18/2, Divide9/2, Divide12/2, Divide15/2  "temp(5)"
  Add14/1 -> Gain14/1
  Product27/1 -> Add14/2, Add13/2, Add12/2
  Subtract2/1 -> Subtract12/2, Product35/2, Product35/1, Add7/2, Gain2/1  "p3real"
  Subtract1/1 -> Subtract11/2, Product36/2, Product36/1, Add6/2, Gain3/1  "p5real"
  Subtract/1 -> Subtract13/2, Product34/1, Product34/2, Add8/2, Gain1/1  "p1real"
  Divide5/1 -> Trigonometric Function1/1
  Constant59/1 -> Product32/2
  Add4/1 -> Subtract9/2  "phase"
  Product30/1 -> Add11/2
  Subtract13/1 -> Product39/2, Product39/1
  Product38/1 -> Add16/1
  Product39/1 -> Add17/1
  Divide21/1 -> a1(1)/1  "a1(1)"
  Product32/1 -> Add16/2, Add10/1, Add13/1
  Subtract7/1 -> Add4/2
  Constant62/1 -> Subtract11/1
  Constant58/1 -> Product32/1
  Divide2/1 -> Trigonometric Function4/1
  Subtract10/1 -> Divide11/1, Divide10/1, Divide9/1  "b0"
  Constant31/1 -> Subtract/1
  Trigonometric Function3/1 -> Subtract6/2
  Product36/1 -> Add14/3
  Add9/1 -> Divide18/1  "a2(5)"
  Product33/1 -> Add9/1, Add15/2, Add14/1
  Constant41/1 -> Add3/2
  Constant44/1 -> Add2/1
  Gain7/1 -> Divide14/1, Divide13/1, Divide12/1  "b1"
  Product35/1 -> Add13/3
  Add16/1 -> Divide22/2, Divide19/2, Divide10/2, Divide13/2, Divide16/2  "temp(3)"
  Constant63/1 -> Subtract12/1
  Divide8/1 -> Subtract10/2, Add5/1, Gain7/1  "rzero"
  Product34/1 -> Add12/3
  Trigonometric Function4/1 -> Subtract7/2
  Trigonometric Function5/1 -> Subtract8/2
  Subtract11/1 -> Product37/2, Product37/1
  Gain11/1 -> Divide21/1  "a1(1)"
  Gain12/1 -> Divide22/1  "a1(3)"
  Constant32/1 -> Subtract1/1
  Trigonometric Function6/1 -> Divide8/2
  Add8/1 -> Product30/2, Product30/1
  Constant40/1 -> Add3/1
  Gain6/1 -> Divide8/1
  Trigonometric Function1/1 -> Subtract7/1
  Add2/1 -> Divide5/1
  Subtract6/1 -> Gain5/1
  Gain13/1 -> Divide23/1  "a1(5)"
  Constant42/1 -> Add2/2
  Divide4/1 -> Trigonometric Function/1
  Product37/1 -> Add15/1
  Gain3/1 -> Divide4/2, Divide1/2
  Divide3/1 -> Trigonometric Function5/1
  Divide1/1 -> Trigonometric Function3/1
  Constant55/1 -> Add8/1
  Divide23/1 -> a1(5)/1  "a1(5)"
  Divide7/1 -> Trigonometric Function6/1
  Add6/1 -> Product29/2, Product29/1
  Product29/1 -> Add9/2
  Constant47/1 -> Subtract9/1
  Constant49/1 -> Subtract10/1
  Trigonometric Function2/1 -> Subtract8/1
  Subtract12/1 -> Product38/2, Product38/1
  Add3/1 -> Divide4/1
  Constant37/1 -> Subtract5/2
  Constant50/1 -> Product27/1
  Add11/1 -> Divide20/1  "a2(1)"
  Subtract5/1 -> Divide3/1
  Add1/1 -> Divide6/1
  Subtract4/1 -> Divide2/1
  Subtract3/1 -> Divide1/1
  Constant34/1 -> Subtract3/1
  Constant45/1 -> Add1/1
  Gain4/1 -> Add4/3
  Constant56/1 -> Product31/1
  Add7/1 -> Product28/2, Product28/1
  Gain5/1 -> Add4/1
  Constant51/1 -> Add5/2
  Product28/1 -> Add10/2
  Divide13/1 -> b1(3)/1  "b1(3)"
  Constant36/1 -> Subtract4/2
  Constant39/1 -> Subtract5/1
  Constant61/1 -> Product33/2
  Constant60/1 -> Product33/1
  Constant54/1 -> Add7/1
  Constant57/1 -> Product31/2
  Constant64/1 -> Subtract13/1
  Add10/1 -> Divide19/1  "a2(3)"
  Constant38/1 -> Subtract4/1
  Trigonometric Function/1 -> Subtract6/1
  Constant35/1 -> Subtract3/2
  Constant43/1 -> Add1/2
  Constant48/1 -> Divide7/2
  Constant53/1 -> Add6/1
  Divide17/1 -> b2(1)/1  "b2(1)"
  Divide12/1 -> b1(5)/1  "b1(5)"
  Divide20/1 -> a2(1)/1  "a2(1)"
  Divide11/1 -> b0(1)/1  "b0(1)"
  Divide14/1 -> b1(1)/1  "b1(1)"
  Divide15/1 -> b2(5)/1  "b2(5)"
  Divide10/1 -> b0(3)/1  "b0(3)"
  Divide22/1 -> a1(3)/1  "a1(3)"
  Divide9/1 -> b0(5)/1  "b0(5)"
  Divide19/1 -> a2(3)/1  "a2(3)"
  Divide16/1 -> b2(3)/1  "b2(3)"
  Gain10/1 -> Gain11/1
  Gain9/1 -> Gain12/1
  Gain14/1 -> Gain13/1

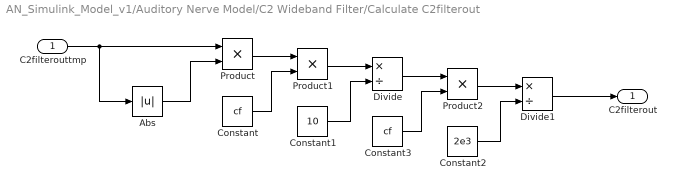
== system AN_Simulink_Model_v1/Auditory Nerve Model/C2 Wideband Filter/Calculate C2filterout ==
  C2filterouttmp : Inport
  Abs : Abs
  Constant : Constant  Value=cf  OutDataTypeStr=single  SampleTime=-1
  Constant1 : Constant  Value=10  OutDataTypeStr=single  SampleTime=-1
  Constant2 : Constant  Value=2e3  OutDataTypeStr=single  SampleTime=-1
  Constant3 : Constant  Value=cf  OutDataTypeStr=single  SampleTime=-1
  Divide : Product  Inputs=*/  SaturateOnIntegerOverflow=on  RndMeth=Zero
  Divide1 : Product  Inputs=*/  SaturateOnIntegerOverflow=on  RndMeth=Zero
  Product : Product
  Product1 : Product
  Product2 : Product
  C2filterout : Outport  VectorParamsAs1DForOutWhenUnconnected=off
  wires:
  C2filterouttmp/1 -> Product/1, Abs/1
  Abs/1 -> Product/2
  Product/1 -> Product1/1
  Constant/1 -> Product1/2
  Product1/1 -> Divide/1
  Constant1/1 -> Divide/2
  Product2/1 -> Divide1/1
  Constant2/1 -> Divide1/2
  Constant3/1 -> Product2/2
  Divide/1 -> Product2/1
  Divide1/1 -> C2filterout/1

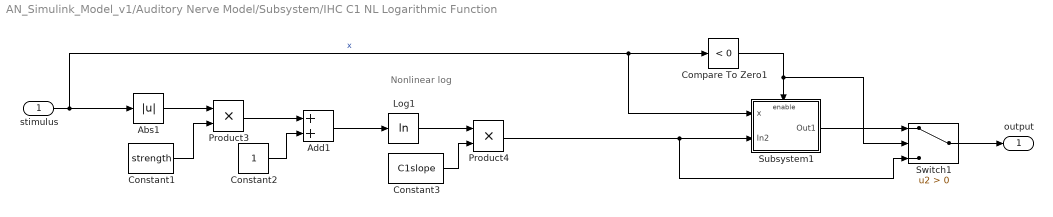
== system AN_Simulink_Model_v1/Auditory Nerve Model/Subsystem/IHC C1 NL Logarithmic Function ==
  note: Nonlinear log
  stimulus : Inport
  Abs1 : Abs
  Add1 : Sum
  Compare To Zero1 : simulink/Logic and Bit Operations/Compare To Zero  relop=<  OutDataTypeStr=boolean
  Constant1 : Constant  Value=strength  OutDataTypeStr=single  SampleTime=-1
  Constant2 : Constant  OutDataTypeStr=single  SampleTime=-1
  Constant3 : Constant  Value=C1slope  OutDataTypeStr=single  SampleTime=-1
  Log1 : Math  Operator=log  SaturateOnIntegerOverflow=on
  Product3 : Product
  Product4 : Product
  Subsystem1 : Subsystem
  Switch1 : Switch  Criteria=u2 > Threshold
  output : Outport  VectorParamsAs1DForOutWhenUnconnected=off
  wires:
  Product3/1 -> Add1/1
  Abs1/1 -> Product3/1
  Subsystem1/1(Out1) -> Switch1/1
  Compare To Zero1/1 -> Subsystem1/Enable, Switch1/2
  Log1/1 -> Product4/1
  Add1/1 -> Log1/1
  Product4/1 -> Switch1/3, Subsystem1/2(In2)
  Switch1/1 -> output/1
  stimulus/1 -> Subsystem1/1(x), Compare To Zero1/1, Abs1/1  "x"
  Constant2/1 -> Add1/2
  Constant3/1 -> Product4/2
  Constant1/1 -> Product3/2

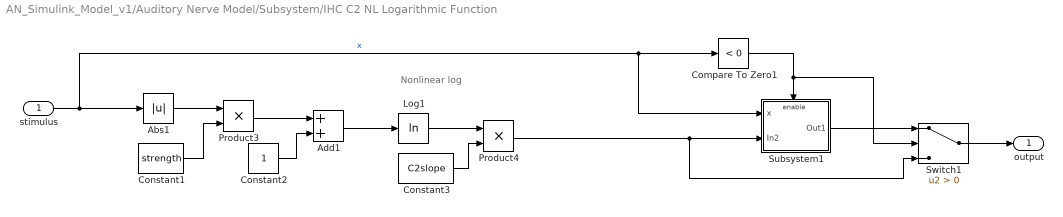
== system AN_Simulink_Model_v1/Auditory Nerve Model/Subsystem/IHC C2 NL Logarithmic Function ==
  note: Nonlinear log
  stimulus : Inport
  Abs1 : Abs
  Add1 : Sum
  Compare To Zero1 : simulink/Logic and Bit Operations/Compare To Zero  relop=<  OutDataTypeStr=boolean
  Constant1 : Constant  Value=strength  OutDataTypeStr=single  SampleTime=-1
  Constant2 : Constant  OutDataTypeStr=single  SampleTime=-1
  Constant3 : Constant  Value=C2slope  OutDataTypeStr=single  SampleTime=-1
  Log1 : Math  Operator=log  SaturateOnIntegerOverflow=on
  Product3 : Product
  Product4 : Product
  Subsystem1 : Subsystem
  Switch1 : Switch  Criteria=u2 > Threshold
  output : Outport  VectorParamsAs1DForOutWhenUnconnected=off
  wires:
  Product3/1 -> Add1/1
  Abs1/1 -> Product3/1
  Subsystem1/1(Out1) -> Switch1/1
  Compare To Zero1/1 -> Subsystem1/Enable, Switch1/2
  Log1/1 -> Product4/1
  Add1/1 -> Log1/1
  Product4/1 -> Switch1/3, Subsystem1/2(In2)
  Switch1/1 -> output/1
  stimulus/1 -> Subsystem1/1(x), Compare To Zero1/1, Abs1/1  "x"
  Constant2/1 -> Add1/2
  Constant3/1 -> Product4/2
  Constant1/1 -> Product3/2

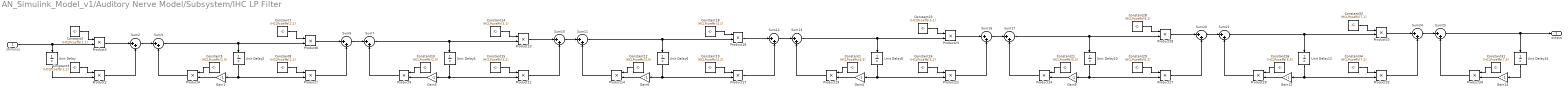
== system AN_Simulink_Model_v1/Auditory Nerve Model/Subsystem/IHC LP Filter ==
  stimulus : Inport  OutDataTypeStr=single
  Constant1 : Constant  Value=IHCLPcoeffs(4,5)  OutDataTypeStr=single  SampleTime=-1
  Constant10 : Constant  Value=IHCLPcoeffs(2,5)  OutDataTypeStr=single  SampleTime=-1
  Constant12 : Constant  Value=IHCLPcoeffs(3,5)  OutDataTypeStr=single  SampleTime=-1
  Constant14 : Constant  Value=IHCLPcoeffs(3,1)  OutDataTypeStr=single  SampleTime=-1
  Constant15 : Constant  Value=IHCLPcoeffs(3,2)  OutDataTypeStr=single  SampleTime=-1
  Constant18 : Constant  Value=IHCLPcoeffs(4,1)  OutDataTypeStr=single  SampleTime=-1
  Constant19 : Constant  Value=IHCLPcoeffs(4,2)  OutDataTypeStr=single  SampleTime=-1
  Constant2 : Constant  Value=IHCLPcoeffs(1,1)  OutDataTypeStr=single  SampleTime=-1
  Constant21 : Constant  Value=IHCLPcoeffs(5,5)  OutDataTypeStr=single  SampleTime=-1
  Constant23 : Constant  Value=IHCLPcoeffs(5,1)  OutDataTypeStr=single  SampleTime=-1
  Constant24 : Constant  Value=IHCLPcoeffs(5,2)  OutDataTypeStr=single  SampleTime=-1
  Constant26 : Constant  Value=IHCLPcoeffs(6,5)  OutDataTypeStr=single  SampleTime=-1
  Constant28 : Constant  Value=IHCLPcoeffs(6,1)  OutDataTypeStr=single  SampleTime=-1
  Constant29 : Constant  Value=IHCLPcoeffs(6,2)  OutDataTypeStr=single  SampleTime=-1
  Constant3 : Constant  Value=IHCLPcoeffs(1,2)  OutDataTypeStr=single  SampleTime=-1
  Constant31 : Constant  Value=IHCLPcoeffs(7,5)  OutDataTypeStr=single  SampleTime=-1
  Constant33 : Constant  Value=IHCLPcoeffs(7,1)  OutDataTypeStr=single  SampleTime=-1
  Constant34 : Constant  Value=IHCLPcoeffs(7,2)  OutDataTypeStr=single  SampleTime=-1
  Constant5 : Constant  Value=IHCLPcoeffs(1,5)  OutDataTypeStr=single  SampleTime=-1
  Constant7 : Constant  Value=IHCLPcoeffs(2,1)  OutDataTypeStr=single  SampleTime=-1
  Constant8 : Constant  Value=IHCLPcoeffs(2,2)  OutDataTypeStr=single  SampleTime=-1
  Gain{1,3..4,6,9,12,14} (7 alike) : Gain  Gain=-1
  Product{2..4,7..9,12..14,17..19,22..24,27..29,32..34} (21 alike) : Product
  Sum{2..3,6..7,10..13,16..17,20..21,24..25} (14 alike) : Sum  Inputs=|++
  Unit Delay{,2,4,6,8,10,12,14} (8 alike) : UnitDelay  SampleTime=-1  HasFrameUpgradeWarning=on
  output : Outport  VectorParamsAs1DForOutWhenUnconnected=off
  wires:
  Unit Delay14/1 -> Gain14/1
  Constant31/1 -> Product34/1
  Product29/1 -> Sum21/2
  Constant33/1 -> Product33/1
  Product13/1 -> Sum10/1
  Product34/1 -> Sum25/2
  Product8/1 -> Sum6/1
  Constant19/1 -> Product17/1
  Gain12/1 -> Product29/2
  Product32/1 -> Sum24/2
  Sum7/1 -> Unit Delay4/1, Product13/2
  Sum21/1 -> Unit Delay12/1, Product33/2
  Sum25/1 -> output/1, Unit Delay14/1
  Gain14/1 -> Product34/2
  Sum24/1 -> Sum25/1
  Product12/1 -> Sum10/2
  Unit Delay2/1 -> Product7/2, Gain1/1
  Unit Delay12/1 -> Product32/2, Gain12/1
  Constant26/1 -> Product29/1
  Product28/1 -> Sum20/1
  Product33/1 -> Sum24/1
  Product19/1 -> Sum13/2
  Product18/1 -> Sum12/1
  Sum16/1 -> Sum17/1
  Product27/1 -> Sum20/2
  Constant34/1 -> Product32/1
  Constant28/1 -> Product28/1
  Unit Delay10/1 -> Product27/2, Gain9/1
  Product24/1 -> Sum17/2
  Unit Delay/1 -> Product2/2
  Sum11/1 -> Unit Delay6/1, Product18/2
  Gain4/1 -> Product19/2
  Constant1/1 -> Product19/1
  stimulus/1 -> Product3/2, Unit Delay/1
  Product4/1 -> Sum3/2
  Constant24/1 -> Product22/1
  Constant21/1 -> Product24/1
  Constant29/1 -> Product27/1
  Gain9/1 -> Product24/2
  Sum20/1 -> Sum21/1
  Sum10/1 -> Sum11/1
  Gain1/1 -> Product4/2
  Unit Delay6/1 -> Product17/2, Gain6/1
  Sum12/1 -> Sum13/1
  Constant15/1 -> Product12/1
  Product14/1 -> Sum11/2
  Unit Delay8/1 -> Product22/2, Gain4/1
  Sum13/1 -> Unit Delay8/1, Product23/2
  Product17/1 -> Sum12/2
  Gain6/1 -> Product14/2
  Constant3/1 -> Product2/1
  Constant8/1 -> Product7/1
  Constant12/1 -> Product14/1
  Product3/1 -> Sum2/1
  Constant14/1 -> Product13/1
  Sum2/1 -> Sum3/1
  Sum17/1 -> Unit Delay10/1, Product28/2
  Product23/1 -> Sum16/1
  Constant10/1 -> Product9/1
  Product9/1 -> Sum7/2
  Constant2/1 -> Product3/1
  Unit Delay4/1 -> Product12/2, Gain3/1
  Product22/1 -> Sum16/2
  Constant18/1 -> Product18/1
  Constant5/1 -> Product4/1
  Constant23/1 -> Product23/1
  Constant7/1 -> Product8/1
  Sum3/1 -> Unit Delay2/1, Product8/2
  Gain3/1 -> Product9/2
  Product2/1 -> Sum2/2
  Sum6/1 -> Sum7/1
  Product7/1 -> Sum6/2

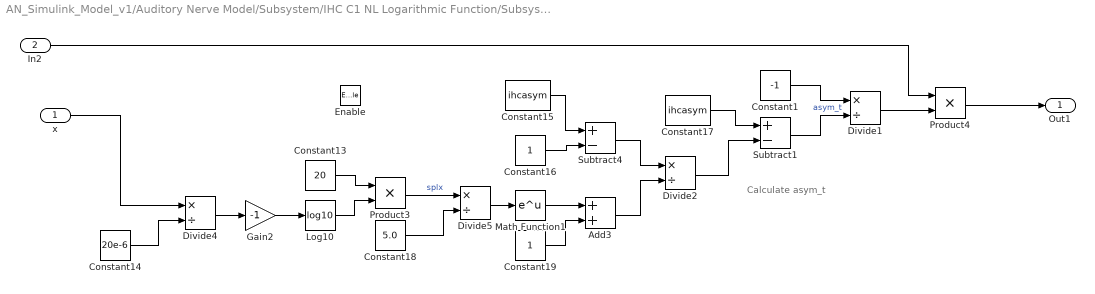
== system AN_Simulink_Model_v1/Auditory Nerve Model/Subsystem/IHC C1 NL Logarithmic Function/Subsystem1 ==
  note: Calculate asym_t
  x : Inport
  In2 : Inport  Port=2
  Enable : EnablePort
  Add3 : Sum
  Constant1 : Constant  Value=-1  OutDataTypeStr=single  SampleTime=-1
  Constant13 : Constant  Value=20  OutDataTypeStr=single  SampleTime=-1
  Constant14 : Constant  Value=20e-6  OutDataTypeStr=single  SampleTime=-1
  Constant15 : Constant  Value=ihcasym  OutDataTypeStr=single  SampleTime=-1
  Constant16 : Constant  OutDataTypeStr=single  SampleTime=-1
  Constant17 : Constant  Value=ihcasym  OutDataTypeStr=single  SampleTime=-1
  Constant18 : Constant  Value=5.0  OutDataTypeStr=single  SampleTime=-1
  Constant19 : Constant  OutDataTypeStr=single  SampleTime=-1
  Divide{1..2,4..5} (4 alike) : Product  Inputs=*/  SaturateOnIntegerOverflow=on  RndMeth=Zero
  Gain2 : Gain  Gain=-1
  Log10 : Math  Operator=log10  SaturateOnIntegerOverflow=on
  Math Function1 : Math  SaturateOnIntegerOverflow=on
  Product3 : Product
  Product4 : Product
  Subtract1 : Sum  Inputs=+-
  Subtract4 : Sum  Inputs=+-
  Out1 : Outport  OutDataTypeStr=single  InitialOutput=[0]
  wires:
  Gain2/1 -> Log10/1
  Constant13/1 -> Product3/1
  Divide5/1 -> Math Function1/1
  Math Function1/1 -> Add3/1
  Product3/1 -> Divide5/1  "splx"
  Constant15/1 -> Subtract4/1
  Log10/1 -> Product3/2
  Constant14/1 -> Divide4/2
  Constant19/1 -> Add3/2
  Divide4/1 -> Gain2/1
  Constant18/1 -> Divide5/2
  Subtract4/1 -> Divide2/1
  Constant17/1 -> Subtract1/1
  Add3/1 -> Divide2/2
  Divide2/1 -> Subtract1/2
  Subtract1/1 -> Divide1/2  "asym_t"
  Constant1/1 -> Divide1/1
  Constant16/1 -> Subtract4/2
  Divide1/1 -> Product4/2
  In2/1 -> Product4/1
  x/1 -> Divide4/1
  Product4/1 -> Out1/1

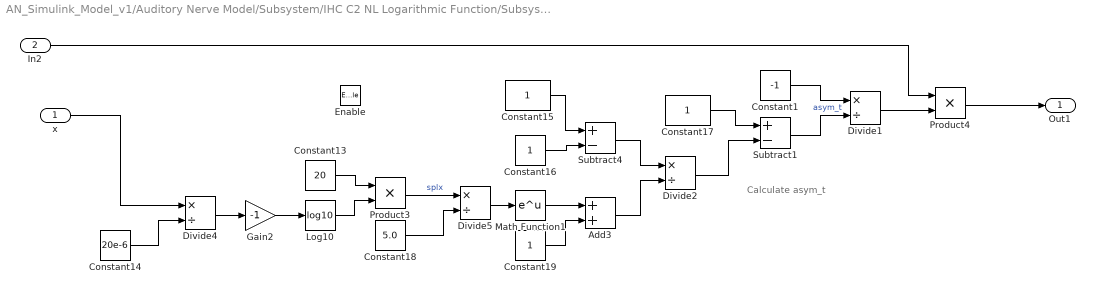
== system AN_Simulink_Model_v1/Auditory Nerve Model/Subsystem/IHC C2 NL Logarithmic Function/Subsystem1 ==
  note: Calculate asym_t
  x : Inport
  In2 : Inport  Port=2
  Enable : EnablePort
  Add3 : Sum
  Constant1 : Constant  Value=-1  OutDataTypeStr=single  SampleTime=-1
  Constant13 : Constant  Value=20  OutDataTypeStr=single  SampleTime=-1
  Constant14 : Constant  Value=20e-6  OutDataTypeStr=single  SampleTime=-1
  Constant{15..17,19} (4 alike) : Constant  OutDataTypeStr=single  SampleTime=-1
  Constant18 : Constant  Value=5.0  OutDataTypeStr=single  SampleTime=-1
  Divide{1..2,4..5} (4 alike) : Product  Inputs=*/  SaturateOnIntegerOverflow=on  RndMeth=Zero
  Gain2 : Gain  Gain=-1
  Log10 : Math  Operator=log10  SaturateOnIntegerOverflow=on
  Math Function1 : Math  SaturateOnIntegerOverflow=on
  Product3 : Product
  Product4 : Product
  Subtract1 : Sum  Inputs=+-
  Subtract4 : Sum  Inputs=+-
  Out1 : Outport  OutDataTypeStr=single  InitialOutput=[0]
  wires:
  Gain2/1 -> Log10/1
  Constant13/1 -> Product3/1
  Divide5/1 -> Math Function1/1
  Math Function1/1 -> Add3/1
  Product3/1 -> Divide5/1  "splx"
  Constant15/1 -> Subtract4/1
  Log10/1 -> Product3/2
  Constant14/1 -> Divide4/2
  Constant19/1 -> Add3/2
  Divide4/1 -> Gain2/1
  Constant18/1 -> Divide5/2
  Subtract4/1 -> Divide2/1
  Constant17/1 -> Subtract1/1
  Add3/1 -> Divide2/2
  Divide2/1 -> Subtract1/2
  Subtract1/1 -> Divide1/2  "asym_t"
  Constant1/1 -> Divide1/1
  Constant16/1 -> Subtract4/2
  Divide1/1 -> Product4/2
  In2/1 -> Product4/1
  x/1 -> Divide4/1
  Product4/1 -> Out1/1
